simulink model "mpc_doubleint_for_speedctrl"  (Simulink 8.2)
settings: Solver=ode45  SolverMode=SingleTasking  StartTime=0.0  StopTime=5  RelTol=1e-3
undefined symbols (not defined in the file): r, x01, x02
libraries: mpclib x1
settings Model: Creator=rchen  LastModifiedBy=leoking99  ExtModeTrigMode=oneshot  ExtModeArmWhenConnect=off
settings DataIOCC: LimitDataPoints=off  SignalLoggingName=sigsOut
settings OptimizationCC: BooleanDataType=off  InitFltsAndDblsToZero=on
settings DebuggingCC: SaveWithParameterizedLinksMsg=none  SignalResolutionControl=TryResolveAllWithWarning  SolverPrmCheckMsg=none  MultiTaskDSMMsg=warning  MultiTaskCondExecSysMsg=none  IntegerOverflowMsg=none
settings HardwareCC: TargetUnknown=on
settings RTWCC: IncludeERTFirstTime=on
settings GRTTargetCC: TargetFcnLib=ansi_tfl_tmw.mat

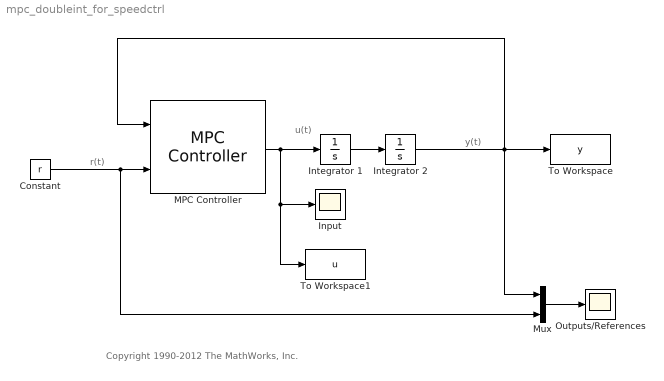
== system mpc_doubleint_for_speedctrl ==
  note: u(t)
  note: y(t)
  note: r(t)
  note: Copyright 1990-2012 The MathWorks, Inc.
  Constant : Constant  Value=r
  Input : Scope
      settings: TimeRange=6  YMin=-1  YMax=1  DataFormat=Structure
  Integrator 1 : Integrator  InitialCondition=x01  UpperSaturationLimit=Inf  LowerSaturationLimit=-Inf
  Integrator 2 : Integrator  InitialCondition=x02  UpperSaturationLimit=Inf  LowerSaturationLimit=-Inf
  MPC Controller : mpclib/MPC Controller  mpcobj=mpc_controller  x0=[]  md_inport=off  mv_inport=off  lims_inport=off  switch_inport=off  ywt_inport=off  duwt_inport=off  rhoeps_inport=off  cost_outport=off  return_sequence=off  return_qpstatus=off  is_multiple=0  enable_value=0  n_mv=1  n_mo=1  n_md=0  n_ts=0.1  is_designfromscratch=0  BlockDataType=double  SampleTimeInherited=off  ref_from_ws=off  ref_signal_name=[]  ref_preview=on  md_from_ws=off  md_signal_name=[]  md_preview=on  from_project=off  project_file=MPCtask.mat
  Mux : Mux  Inputs=2
  Outputs/References : Scope
      settings: TimeRange=5  YMin=0  YMax=1.5  DataFormat=Structure
  To Workspace : ToWorkspace  VariableName=y  SampleTime=-1
      settings: MaxDataPoints=Inf
  To Workspace1 : ToWorkspace  VariableName=u  SampleTime=-1
      settings: MaxDataPoints=Inf
  wires:
  MPC Controller/1 -> Integrator 1/1, Input/1, To Workspace1/1
  Integrator 2/1 -> Mux/1, MPC Controller/1, To Workspace/1
  Mux/1 -> Outputs/References/1
  Constant/1 -> MPC Controller/2, Mux/2
  Integrator 1/1 -> Integrator 2/1
